simulink model "observador1"  (R2013a)
settings: Solver=ode45  StartTime=0.0  StopTime=1  RelTol=1e-3
values from neighbouring files (symbols this model uses):
  a = double(a)    [SAd.m]    (also in ackerobs.m = poly(p); distanciaeuclidiana.m; ejercisiou3diff.m = pinv(ci); ejmvallesypicos.m = imread('cameraman.tif','tif'))
  b = C*G^(i-1)    [ackerobs.m]    (also in espcolor.m = double(b); firttf.m = [1 0 -2];freqz(a,b))
  c = impixel()    [SAd.m]    (also in distanciaeuclidiana.m; ejercisiou3diff.m = simplify(C))
  L = phi*inv(N)*[zeros(n-2,1);1]    [ackerobs.m]
libraries: powerlib x10
settings Model: Creator=Daniel  LastModifiedBy=Daniel

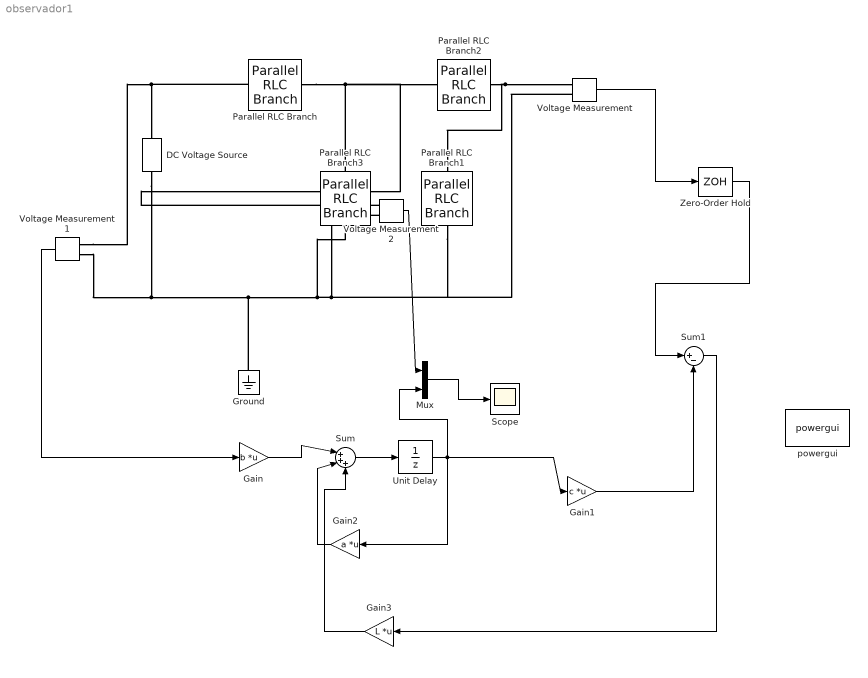
== system observador1 ==
  DC Voltage Source : powerlib/Electrical Sources/DC Voltage Source  Amplitude=1  Measurements=None
  Gain : Gain  Gain=b  Multiplication=Matrix(K*u) (u vector)
  Gain1 : Gain  Gain=c  Multiplication=Matrix(K*u) (u vector)
  Gain2 : Gain  Gain=a  Multiplication=Matrix(K*u) (u vector)
  Gain3 : Gain  Gain=L  Multiplication=Matrix(K*u) (u vector)
  Ground : powerlib/Elements/Ground  LConnTagsString=a
  Mux : Mux  Inputs=2
  Parallel RLC Branch : powerlib/Elements/Parallel RLC Branch  LConnTagsString=a  RConnTagsString=__new0  BranchType=R  Resistance=10000  Inductance=1e-3  SetiL0=off  InitialCurrent=0  Capacitance=1e-6  Setx0=off  InitialVoltage=0  Measurements=None
  Parallel RLC Branch1 : powerlib/Elements/Parallel RLC Branch  LConnTagsString=a  RConnTagsString=__new0  BranchType=C  Resistance=1  Inductance=1e-3  SetiL0=off  InitialCurrent=0  Capacitance=10e-6  Setx0=off  InitialVoltage=0  Measurements=None
  Parallel RLC Branch2 : powerlib/Elements/Parallel RLC Branch  LConnTagsString=a  RConnTagsString=__new0  BranchType=R  Resistance=10000  Inductance=1e-3  SetiL0=off  InitialCurrent=0  Capacitance=1e-6  Setx0=off  InitialVoltage=0  Measurements=None
  Parallel RLC Branch3 : powerlib/Elements/Parallel RLC Branch  LConnTagsString=a  RConnTagsString=__new0  BranchType=C  Resistance=1  Inductance=1e-3  SetiL0=off  InitialCurrent=0  Capacitance=10e-6  Setx0=off  InitialVoltage=0  Measurements=None
  Scope : Scope
  Sum : Sum  Inputs=|+++
  Sum1 : Sum  Inputs=|+-
  Unit Delay : UnitDelay  InitialCondition=.001  SampleTime=.001
  Voltage Measurement : powerlib/Measurements/Voltage Measurement  PhasorSimulation=off  OutputType=Complex  PSBequivalent=0
  Voltage Measurement1 : powerlib/Measurements/Voltage Measurement  PhasorSimulation=off  OutputType=Complex  PSBequivalent=0
  Voltage Measurement2 : powerlib/Measurements/Voltage Measurement  PhasorSimulation=off  OutputType=Complex  PSBequivalent=0
  Zero-Order Hold : ZeroOrderHold  SampleTime=.001
  powergui : powerlib/powergui  Priority=1  SimulationMode=Continuous  SolverType=Tustin  SampleTime=50e-6  frequency=60  SPID=off  DisableSnubberDevices=off  DisableRonSwitches=off  DisableVfSwitches=off  SwTol=0  Interpol=off  DisplayEquations=off  frequencyindice=0  Pbase=100e6  ErrMax=1e-4  Iterations=50  UnitsV=kV  UnitsW=MW  FunctionMessages=off  echomessages=off  HookPort=off  EnableUseOfTLC=off  x0status=blocks  RestoreLinks=warning  ResistiveCurrentMeasurement=off  Frange=[0:2:500]  Ylog=off  Xlog=on  ShowGrid=off  save=off  variable=ZData  ZoomFFT=off  StartTime=0.0  cycles=1  DisplayStyle=1  fundamental=60  FreqAxis=off  MaxFrequency=1000  frequencyindicesteady=1  RmsSteady=1  display=off  Ts=0  methode=off
  wires:
  Sum/1 -> Unit Delay/1
  Gain2/1 -> Sum/2
  Gain/1 -> Sum/1
  Unit Delay/1 -> Mux/2, Gain2/1, Gain1/1
  Voltage Measurement/1 -> Zero-Order Hold/1
  Gain1/1 -> Sum1/2
  Voltage Measurement1/1 -> Gain/1
  Sum1/1 -> Gain3/1
  Gain3/1 -> Sum/3
  Zero-Order Hold/1 -> Sum1/1
  Voltage Measurement2/1 -> Mux/1
  Mux/1 -> Scope/1
  connections:
  Parallel RLC Branch/LConn1 -- Voltage Measurement1/LConn1 -- DC Voltage Source/RConn1
  DC Voltage Source/LConn1 -- Voltage Measurement1/LConn2 -- Parallel RLC Branch1/RConn1 -- Voltage Measurement/LConn2 -- Voltage Measurement2/LConn2 -- Parallel RLC Branch3/RConn1 -- Ground/LConn1
  Parallel RLC Branch/RConn1 -- Voltage Measurement2/LConn1 -- Parallel RLC Branch2/LConn1 -- Parallel RLC Branch3/LConn1
  Parallel RLC Branch2/RConn1 -- Voltage Measurement/LConn1 -- Parallel RLC Branch1/LConn1
